simulink model "minipro"  (R2021a)
settings: Solver=VariableStepAuto  StartTime=0.0  StopTime=5  RelTol=1e-3
values from neighbouring files (symbols this model uses):
  Left_Turn_AngularLimit = -120.0    [minipro_sldd.sldd]
  LeftTurn_RoadSign = -120.0    [minipro_sldd.sldd]
  Right_Turn_AngularLimit = 30.0    [minipro_sldd.sldd]
  RightTurn_RoadSign = 30.0    [minipro_sldd.sldd]
  Straight_Drive_Steering_Angle = 0.0    [minipro_sldd.sldd]
  Straight_RoadSign = 0.0    [minipro_sldd.sldd]
libraries: simulink x3
settings Model: DataDictionary=minipro_sldd.sldd  Creator=vviswanathan  LastModifiedBy=vviswanathan

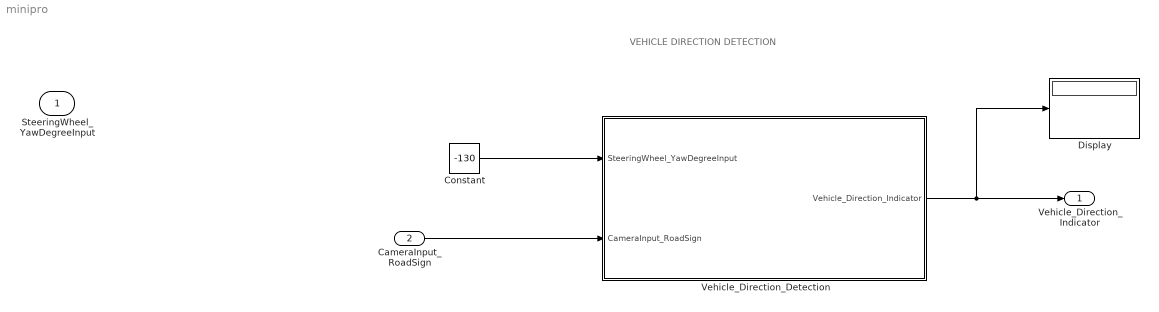
== system minipro ==
  note: VEHICLE DIRECTION DETECTION
  SteeringWheel_YawDegreeInput : Inport
  CameraInput_RoadSign : Inport  Port=2
  Constant : Constant  Value=-130
  Display : Display
  Vehicle_Direction_Detection : Subsystem
  Vehicle_Direction_Indicator : Outport  SignalName=Vehicle_Direction_Indicator
  wires:
  CameraInput_RoadSign/1 -> Vehicle_Direction_Detection/2(CameraInput_RoadSign)
  Vehicle_Direction_Detection/1(Vehicle_Direction_Indicator) -> Display/1, Vehicle_Direction_Indicator/1
  Constant/1 -> Vehicle_Direction_Detection/1(SteeringWheel_YawDegreeInput)

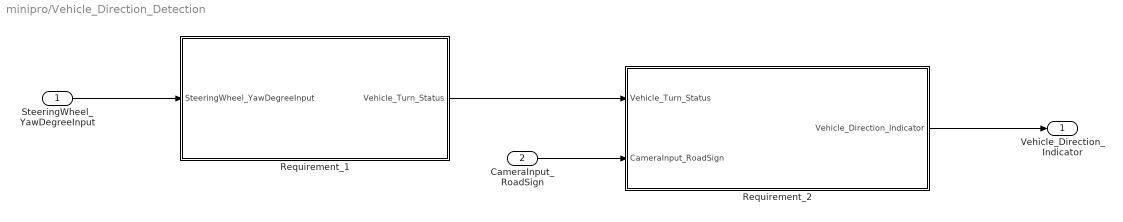
== system minipro/Vehicle_Direction_Detection ==
  SteeringWheel_YawDegreeInput : Inport
  CameraInput_RoadSign : Inport  Port=2
  Requirement_1 : Subsystem
  Requirement_2 : Subsystem
  Vehicle_Direction_Indicator : Outport
  wires:
  CameraInput_RoadSign/1 -> Requirement_2/2(CameraInput_RoadSign)
  SteeringWheel_YawDegreeInput/1 -> Requirement_1/1(SteeringWheel_YawDegreeInput)
  Requirement_1/1(Vehicle_Turn_Status) -> Requirement_2/1(Vehicle_Turn_Status)
  Requirement_2/1(Vehicle_Direction_Indicator) -> Vehicle_Direction_Indicator/1

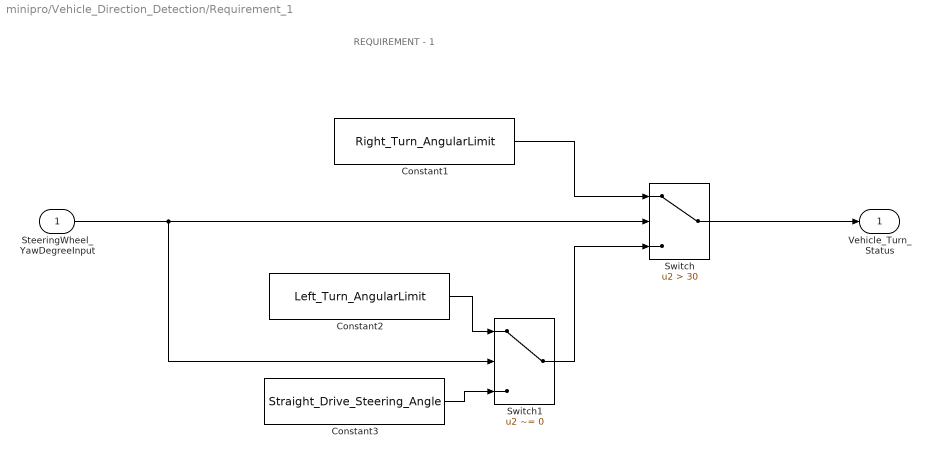
== system minipro/Vehicle_Direction_Detection/Requirement_1 ==
  note: REQUIREMENT - 1
  SteeringWheel_YawDegreeInput : Inport
  Constant1 : Constant  Value=Right_Turn_AngularLimit
  Constant2 : Constant  Value=Left_Turn_AngularLimit
  Constant3 : Constant  Value=Straight_Drive_Steering_Angle
  Switch : Switch  Criteria=u2 > Threshold  Threshold=30
  Switch1 : Switch  Criteria=u2 ~= 0
  Vehicle_Turn_Status : Outport
  wires:
  Switch/1 -> Vehicle_Turn_Status/1
  SteeringWheel_YawDegreeInput/1 -> Switch1/2, Switch/2
  Constant3/1 -> Switch1/3
  Constant1/1 -> Switch/1
  Switch1/1 -> Switch/3
  Constant2/1 -> Switch1/1

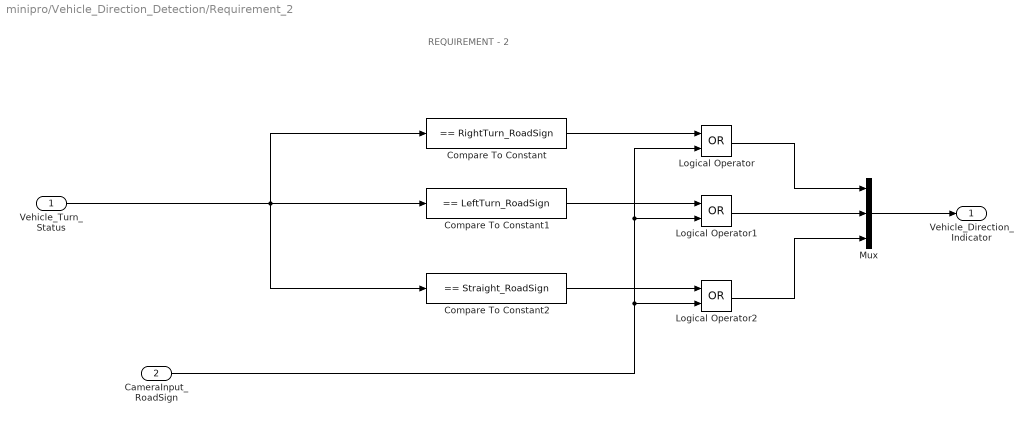
== system minipro/Vehicle_Direction_Detection/Requirement_2 ==
  note: REQUIREMENT - 2
  Vehicle_Turn_Status : Inport
  CameraInput_RoadSign : Inport  Port=2
  Compare To Constant : simulink/Logic and Bit Operations/Compare To Constant  relop===  const=RightTurn_RoadSign  OutDataTypeStr=boolean
  Compare To Constant1 : simulink/Logic and Bit Operations/Compare To Constant  relop===  const=LeftTurn_RoadSign  OutDataTypeStr=boolean
  Compare To Constant2 : simulink/Logic and Bit Operations/Compare To Constant  relop===  const=Straight_RoadSign  OutDataTypeStr=boolean
  Logical Operator : Logic  Operator=OR  AllPortsSameDT=off  OutDataTypeStr=boolean
  Logical Operator1 : Logic  Operator=OR  AllPortsSameDT=off  OutDataTypeStr=boolean
  Logical Operator2 : Logic  Operator=OR  AllPortsSameDT=off  OutDataTypeStr=boolean
  Mux : Mux  Inputs=3
  Vehicle_Direction_Indicator : Outport
  wires:
  Vehicle_Turn_Status/1 -> Compare To Constant2/1, Compare To Constant1/1, Compare To Constant/1
  Logical Operator1/1 -> Mux/2
  Compare To Constant/1 -> Logical Operator/1
  CameraInput_RoadSign/1 -> Logical Operator/2, Logical Operator1/2, Logical Operator2/2
  Logical Operator/1 -> Mux/1
  Logical Operator2/1 -> Mux/3
  Mux/1 -> Vehicle_Direction_Indicator/1
  Compare To Constant1/1 -> Logical Operator1/1
  Compare To Constant2/1 -> Logical Operator2/1
